simulink model "Ejercicio2_09_03_172222"  (R2013a)
settings: Solver=ode45  StartTime=0.0  StopTime=10.0  RelTol=1e-3
libraries: powerlib x8
settings Model: Creator=Miguel  LastModifiedBy=Miguel

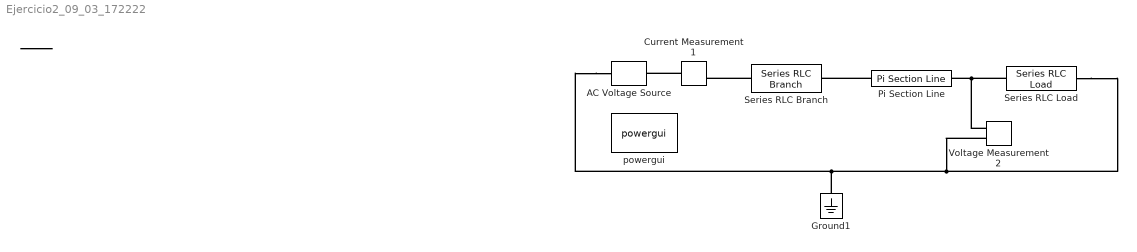
== system Ejercicio2_09_03_172222 ==
  AC Voltage Source : powerlib/Electrical Sources/AC Voltage Source  Amplitude=114588.6594*sqrt(2)  Phase=1.795612043  Frequency=60  SampleTime=0  Measurements=Voltage
  Current Measurement1 : powerlib/Measurements/Current Measurement  PhasorSimulation=on  OutputType=Complex  PSBequivalent=0
  Ground1 : powerlib/Elements/Ground  LConnTagsString=a
  Pi Section Line : powerlib/Elements/Pi Section Line  LConnTagsString=__new0  RConnTagsString=__new0  Frequency=60  Resistance=0.2  Inductance=0.43/(2*pi*60)  Capacitance=2.6e-6/(2*pi*60)  Length=60  PiSections=1  Measurements=None
      settings: AttributesFormatString=\n
  Series RLC Branch : powerlib/Elements/Series RLC Branch  LConnTagsString=__new0  RConnTagsString=__new0  BranchType=L  Resistance=1  Inductance=1e-9  SetiL0=off  InitialCurrent=0  Capacitance=1e-6  Setx0=off  InitialVoltage=0  Measurements=None
  Series RLC Load : powerlib/Elements/Series RLC Load  LConnTagsString=a  RConnTagsString=__new0  NominalVoltage=110e3  NominalFrequency=60  ActivePower=20e6  InductivePower=10e6  CapacitivePower=0  Setx0=off  InitialVoltage=0  SetiL0=off  InitialCurrent=0  Measurements=None
  Voltage Measurement2 : powerlib/Measurements/Voltage Measurement  PhasorSimulation=on  OutputType=Complex  PSBequivalent=0
  powergui : powerlib/powergui  Priority=1  SimulationMode=Phasor  SolverType=Tustin  SampleTime=50e-6  frequency=60  SPID=off  DisableSnubberDevices=off  DisableRonSwitches=off  DisableVfSwitches=off  SwTol=0  Interpol=off  DisplayEquations=off  frequencyindice=60  Pbase=100e6  ErrMax=1e-4  Iterations=50  UnitsV=kV  UnitsW=MW  FunctionMessages=off  echomessages=off  HookPort=off  EnableUseOfTLC=off  x0status=blocks  RestoreLinks=warning  ResistiveCurrentMeasurement=off  Frange=[0:2:500]  Ylog=off  Xlog=on  ShowGrid=off  save=off  variable=ZData  ZoomFFT=off  StartTime=0.0  cycles=1  DisplayStyle=1  fundamental=60  FreqAxis=off  MaxFrequency=1000  frequencyindicesteady=1  RmsSteady=2  display=off  Ts=0  methode=off
  connections:
  ?
  Pi Section Line/LConn1 -- Series RLC Branch/RConn1
  Pi Section Line/RConn1 -- Series RLC Load/LConn1 -- Voltage Measurement2/LConn1
  AC Voltage Source/LConn1 -- Series RLC Load/RConn1 -- Voltage Measurement2/LConn2 -- Ground1/LConn1
  Series RLC Branch/LConn1 -- Current Measurement1/RConn1
  Current Measurement1/LConn1 -- AC Voltage Source/RConn1
